simulink model "simulacion_v1"  (R2021b)
settings: Solver=VariableStepAuto  StartTime=0.0  StopTime=100  RelTol=1e-3
undefined symbols (not defined in the file or in its folder): F, h, km, Light, m, MIL, Moderate, s, sigbuilder_block
libraries: slpidlib x19, simulink x18, simulink_extras x15, aerolibconvert2 x4, aerolibwind2 x3, shared6dof x1, sharedtransform x1, sim3dlib x1, uavsim3dlib x1
(part 1 of 3)
settings Model: PacingRate=0.710000  Creator=luisq  LastModifiedBy=luisq
settings SolverCC: AlgebraicLoopSolver=TrustRegion
settings DebuggingCC: SFMachineParentedDataDiag=warning

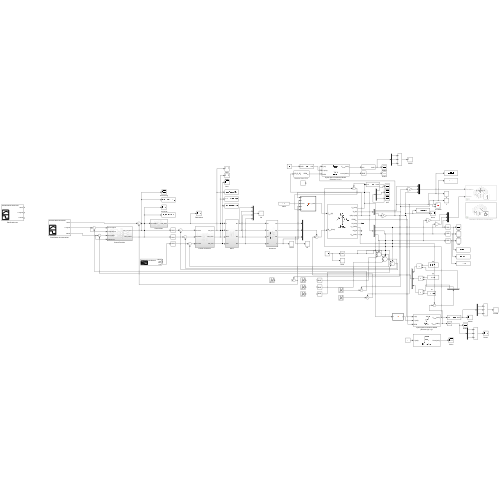
[thumbnail: Simulink's stored preview of the top-level diagram]
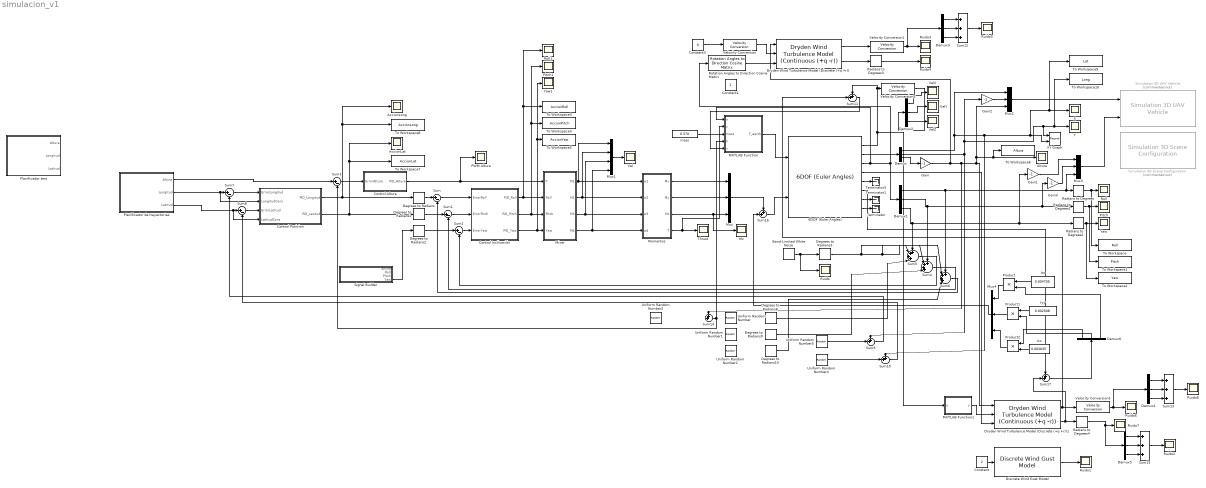
== system simulacion_v1 ==
  6DOF (Euler Angles) : shared6dof/6DOF (Euler Angles)  units=Metric (MKS)  mtype=Fixed  rep=Euler Angles  xme_0=[0 0 0]  Vm_0=[0 0 0]  eul_0=[0 0 0]  pm_0=[0 0 0]  mass_0=0.570  mass_e=0.5  mass_f=2.0  inertia=[0.002635 0 0; 0 0.002508 0; 0 0 0.004705]  inertia_e=eye(3)  inertia_f=2*eye(3)  k_quat=1.0  vre_flag=on  abi_flag=off  aMode=0  xme_statename=''  Vm_statename=''  eul_statename=''  quat_statename=''  pm_statename=''  mass_statename=''
      settings: SourceProductBaseCode=AE,PW,DR,MT,UV,VE
  AccionLat : Scope
  AccionLong : Scope
  Altura : Scope
  Band-Limited White Noise : simulink/Sources/Band-Limited White Noise  Cov=[0.00005]  Ts=0.006  seed=[1165241]
  Constant : Constant  Value=2
  Constant1 : Constant
  Constant3 : Constant  Value=0
  Control Altura : Subsystem
  Control Inclinación : Subsystem
  Control Posicion : Subsystem
  Degrees to Radians{,1..3,8..10} (7 alike) : simulink_extras/Transformations/Degrees to Radians
  Demux{,1..6} (7 alike) : Demux  Outputs=3
  Discrete Wind Gust Model : aerolibwind2/Discrete Wind Gust Model  units=Metric (MKS)  Gx=on  Gy=on  Gz=on  t_0=1  d_m=[100 100 100]  v_m=[2 2 2]
  Dryden Wind Turbulence Model (Discrete (+q +r)) : aerolibwind2/Dryden Wind Turbulence Model  (Continuous (+q -r))  units=Metric (MKS)  spec=MIL-F-8785C  model=Discrete Dryden (+q +r)  W20=15  Wdeg=0  TurbProb=10^-2 - Light  L_high=533.4  Wingspan=10  ts=0.1  Seed=[2753 27856 45178 58756]  T_on=on
  Dryden Wind Turbulence Model (Discrete (+q +r))1 : aerolibwind2/Dryden Wind Turbulence Model  (Continuous (+q -r))  units=Metric (MKS)  spec=MIL-F-8785C  model=Discrete Dryden (+q +r)  W20=1  Wdeg=0  TurbProb=10^-3 - Moderate  L_high=10  Wingspan=20  ts=0.1  Seed=[2753 27856 45178 58756]  T_on=on
  Gain{,1..3} (4 alike) : Gain  Gain=-1
  Ixx : Constant  Value=0.002635
  Iyy : Constant  Value=0.002508
  Izz : Constant  Value=0.004705
  MATLAB Function : MATLAB Function  TreatAsAtomicUnit=on
  MATLAB Function1 : MATLAB Function  TreatAsAtomicUnit=on
  "Mixer " : Subsystem
  Momentos : Subsystem
  Mux{,2..4} (4 alike) : Mux  Inputs=3
  Mux1 : Mux
  Mz : Scope
  PWM Altura : Scope
  Pitch : Scope
  Pitch1 : Scope
  Planificador de trayectorias : Subsystem  Tag=STV Subsys  LoadFcn=sigbuilder_block('load');  StartFcn=sigbuilder_block('start');  StopFcn=sigbuilder_block('stop');  ClipboardFcn=sigbuilder_block('clipboard');  mask(Sigbuilder block){tuvar=[0:10]}
      mask help: Simulink:masks:SigbuilderBlock_MD
      mask init:
      | if ~strcmp(get_param(bdroot(gcbh),'SimulationStatus'),'stopped') tuvar = sigbuilder_block('maskInit'); end
      settings: CopyFcn=sigbuilder_block('copy');  DeleteFcn=sigbuilder_block('delete');  ModelCloseFcn=sigbuilder_block('modelClose');  PreSaveFcn=sigbuilder_block('preSave');  PauseFcn=sigbuilder_block('pause');  ContinueFcn=sigbuilder_block('continue');  NameChangeFcn=sigbuilder_block('namechange');  OpenFcn=sigbuilder_block('open',[438 258 412.5 377.25 ]);  CloseFcn=sigbuilder_block('close');
      mask Display: plot(0, 0, 100, 100,[2, 2, 32, 32, 2], [68, 8, 8, 68, 68],[32, 2], [38, 38], [32, 19, 2],[53, 60, 44], [32, 17, 17, 2],[16, 16, 31, 31]);txt = getActiveGroup(gcbh);text(2, 100, txt,'verticalAlignment', 'top');
  Planificador test : Subsystem  Tag=STV Subsys  LoadFcn=sigbuilder_block('load');  StartFcn=sigbuilder_block('start');  StopFcn=sigbuilder_block('stop');  ClipboardFcn=sigbuilder_block('clipboard');  mask(Sigbuilder block){tuvar=[0:10]}
      mask help: Simulink:masks:SigbuilderBlock_MD
      mask init:
      | if ~strcmp(get_param(bdroot(gcbh),'SimulationStatus'),'stopped') tuvar = sigbuilder_block('maskInit'); end
      settings: CopyFcn=sigbuilder_block('copy');  DeleteFcn=sigbuilder_block('delete');  ModelCloseFcn=sigbuilder_block('modelClose');  PreSaveFcn=sigbuilder_block('preSave');  PauseFcn=sigbuilder_block('pause');  ContinueFcn=sigbuilder_block('continue');  NameChangeFcn=sigbuilder_block('namechange');  OpenFcn=sigbuilder_block('open',[438 258 412.5 377.25 ]);  CloseFcn=sigbuilder_block('close');
      mask Display: plot(0, 0, 100, 100,[2, 2, 32, 32, 2], [68, 8, 8, 68, 68],[32, 2], [38, 38], [32, 19, 2],[53, 60, 44], [32, 17, 17, 2],[16, 16, 31, 31]);txt = getActiveGroup(gcbh);text(2, 100, txt,'verticalAlignment', 'top');
  Product : Product
  Product1 : Product
  Product2 : Product
  Radians to Degrees{,1..4} (5 alike) : simulink_extras/Transformations/Radians to Degrees
  Roll : Scope
  Roll1 : Scope
  Rotation Angles to Direction Cosine Matrix : sharedtransform/Rotation Angles to Direction Cosine Matrix  rotationOrder=ZYX  aMode=aMode
      settings: SourceProductBaseCode=AE,PW,DR,MT,UV,VE
  Ruido{,1..8} (9 alike) : Scope
  Signal Builder : Subsystem  Tag=STV Subsys  LoadFcn=sigbuilder_block('load');  StartFcn=sigbuilder_block('start');  StopFcn=sigbuilder_block('stop');  ClipboardFcn=sigbuilder_block('clipboard');  mask(Sigbuilder block){tuvar=[0:10]}
      mask help: Simulink:masks:SigbuilderBlock_MD
      mask init:
      | if ~strcmp(get_param(bdroot(gcbh),'SimulationStatus'),'stopped') tuvar = sigbuilder_block('maskInit'); end
      settings: CopyFcn=sigbuilder_block('copy');  DeleteFcn=sigbuilder_block('delete');  ModelCloseFcn=sigbuilder_block('modelClose');  PreSaveFcn=sigbuilder_block('preSave');  PauseFcn=sigbuilder_block('pause');  ContinueFcn=sigbuilder_block('continue');  NameChangeFcn=sigbuilder_block('namechange');  OpenFcn=sigbuilder_block('open',[665.25 86.25 550.5 399.75 ]);  CloseFcn=sigbuilder_block('close');
      mask Display: plot(0, 0, 100, 100,[2, 2, 32, 32, 2], [68, 8, 8, 68, 68],[32, 2], [38, 38], [32, 19, 2],[53, 60, 44], [32, 17, 17, 2],[16, 16, 31, 31]);txt = getActiveGroup(gcbh);text(2, 100, txt,'verticalAlignment', 'top');
  Simulation 3D Scene Configuration : sim3dlib/Simulation 3D Scene Configuration  Priority=0  Commented=on  ProjectFormat_internal=Default Scenes  ProjectFormat=Default Scenes  SceneDesc=US city block  ProjectName=G:\MATLAB\R2021b\toolbox\shared\sim3d_projects\automotive_project\UE4\WindowsNoEditor\VehicleSimulation.exe  ScenePath=/Game/Maps/USCityBlock  vehTagList={'Scene Origin';'SimulinkVehicle1'}  vehTag=SimulinkVehicle1  OpVisEn=off  Ts=1/60  EnableWindow=on  EnableWeather=off  SunAltitude=40.0  SunAzimuth=90  clouds=10  wind=1  fog=0  rain=0  sensorTag=MainCamera1  sensorId=1  sensorName=MainCamera1  mountLoc=Origin  offsetFlag=off  tmountOffset=[0, 0, 0]  rmountOffset=[0, 0, 0]  HorizontalResolution=1280  VerticalResolution=720  HorizontalFOV=60  mountPoint=[0 0 0]  mountOrientation=[0 0 0]  aMode=4  ID=1
      settings: SourceProductBaseCode=AE,DR,UV,VE
  Simulation 3D UAV Vehicle : uavsim3dlib/Simulation 3D UAV Vehicle  Priority=-1  Commented=on  Mesh=Quadrotor  MeshPath=/MathWorksUAVContent/UAVs/HexaRotorUAV/HexaRotor.HexaRotor  Color=Black  ActorName=SimulinkVehicle1  InitialTranslation=[0 0 0]  InitialRotation=[0 0 0]  SampleTime=-1  ActorType=SimulinkVehicle  ID=1  aMode=4  ActorTag=SimulinkVehicle1
      settings: SourceProductBaseCode=UV
  Sum{,1..3,7..8} (6 alike) : Sum  Inputs=|+-
  Sum{9..11,14,16..17} (6 alike) : Sum  Inputs=++|
  Sum12 : Sum  Inputs=+++
  Sum13 : Sum  Inputs=+++
  Sum15 : Sum  Inputs=+++
  Sum4 : Sum  Inputs=++++|
  Sum5 : Sum  Inputs=++++|
  Sum6 : Sum  Inputs=++++|
  Terminator : Terminator
  Terminator1 : Terminator
  Terminator3 : Terminator
  Thrust : Scope
  To Workspace : ToWorkspace  VariableName=Roll  SaveFormat=Timeseries  SampleTime=-1
  To Workspace1 : ToWorkspace  VariableName=Pitch  SaveFormat=Timeseries  SampleTime=-1
  To Workspace10 : ToWorkspace  VariableName=Long  SaveFormat=Timeseries  SampleTime=-1
  To Workspace2 : ToWorkspace  VariableName=Yaw  SaveFormat=Timeseries  SampleTime=-1
  To Workspace3 : ToWorkspace  VariableName=AccionRoll  SaveFormat=Timeseries  SampleTime=-1
  To Workspace4 : ToWorkspace  VariableName=AccionPitch  SaveFormat=Timeseries  SampleTime=-1
  To Workspace5 : ToWorkspace  VariableName=AccionYaw  SaveFormat=Timeseries  SampleTime=-1
  To Workspace6 : ToWorkspace  VariableName=Altura  SaveFormat=Timeseries  SampleTime=-1
  To Workspace7 : ToWorkspace  VariableName=AccionLat  SaveFormat=Timeseries  SampleTime=-1
  To Workspace8 : ToWorkspace  VariableName=AccionLong  SaveFormat=Timeseries  SampleTime=-1
  To Workspace9 : ToWorkspace  VariableName=Lat  SaveFormat=Timeseries  SampleTime=-1
  Uniform Random Number : UniformRandomNumber  Minimum=-2.5  Maximum=2.5  Seed=17864  SampleTime=0.006
  Uniform Random Number1 : UniformRandomNumber  Minimum=-2.5  Maximum=2.5  Seed=78834537  SampleTime=0.006
  Uniform Random Number2 : UniformRandomNumber  Minimum=-2.5  Maximum=2.5  Seed=2564558  SampleTime=0.006
  Uniform Random Number3 : UniformRandomNumber  Minimum=-0.6  Maximum=0.6  Seed=418765  SampleTime=0.006
  Uniform Random Number4 : UniformRandomNumber  Minimum=-0.01  Maximum=0.01  Seed=48576  SampleTime=0.006
  Uniform Random Number5 : UniformRandomNumber  Minimum=-0.01  Maximum=0.01  Seed=184832  SampleTime=0.006
  Vel : Scope
  VelX : Scope
  VelY : Scope
  VelZ : Scope
  Velocity Conversion : aerolibconvert2/Velocity Conversion  IU=km/h  OU=m/s
  Velocity Conversion1 : aerolibconvert2/Velocity Conversion  IU=m/s  OU=km/h
  Velocity Conversion3 : aerolibconvert2/Velocity Conversion  IU=m/s  OU=km/h
  Velocity Conversion5 : aerolibconvert2/Velocity Conversion  IU=m/s  OU=km/h
  X : Scope
  XY Graph : Record  FileSettingsInternal="{\"entries\":[{\"content\":{\"excelSettings\":{\"content\":{},\"type\":\"Streamout.ExcelSettings\"}},\"type\":\"Streamout.FileSettingStorage\",\"uuid\":\"2a93f9ce-f61f-4d98-8c9f-4a9fc70b4bb0\"}],\"packageUris\":[\"http://schema.mathworks.com/mf0/streamout_blocks/R2020a\"],\"version\":\"1.0\"}"  Layout=[1 1]  SignalsInternal="{\"entries\":[{\"content\":{\"signals\":[{\"content\":{\"blockPath\":[\"simulacion_v1/XY Graph\"],\"channel\":[],\"dimensions\":[1],\"domain\":\"simulacion_v1/XY Graph\",\"lineColor\":\"#0072bd\",\"plots\":[],\"port\":1,\"sid\":[\"\"],\"signalID\":535,\"signalName\":\"Demux:2\"},\"type\":\"RecordBlkView.Signal\",\"uuid\":\"45a79901-b02e-4be6-b1bb-67b95a6d7ae1\"},{\"content\":{\"blockPath\":[\"simulacion_v1/XY Graph\"],\"channel\":[],\"dimensions\":[1],\"domain\":\"simulacion_v1/XY Graph\",\"lineColor\":\"#d95319\",\"plots\":[],\"port\":2,\"sid\":[\"\"],\"signalID\":539,\"signalName\":\"Demux:1\"},\"type\":\"RecordBlkView.Signal\",\"uuid\":\"d0057eb7-e3a9-49c5-b525-a3b9d954fb19\"}]},\"type\":\"RecordBlkView.InputSignals\",\"uuid\":\"e3ca6051-dc1f-4f56-a0fa-706f4109eb97\"}],\"packageUris\":[\"http://schema.mathworks.com/mf0/streamout_blocks/R2020a\"],\"version\":\"1.0\"}"  CompatibilityTag=XY  st=0.5
  Y : Scope
  Yaw : Scope
  Yaw1 : Scope
  "mass " : Constant  Value=0.570
  wires:
  MATLAB Function/1(F_earth) -> 6DOF (Euler Angles)/1
  Momentos/1(Mx) -> Mux/1
  Momentos/3("Mz ") -> Mz/1, Mux/3
  Momentos/2("My ") -> Mux/2
  "mass "/1 -> MATLAB Function/3(mass)
  6DOF (Euler Angles)/3 -> Demux1/1, Rotation Angles to Direction Cosine Matrix/1, MATLAB Function/1(u)
  6DOF (Euler Angles)/2 -> Demux/1
  Demux/2 -> Sum9/1, XY Graph/1, To Workspace10/1, Y/1, Gain2/1
  Momentos/4(T) -> Thrust/1, MATLAB Function/2(c)
  Demux/3 -> Gain/1
  Demux1/1 -> Sum6/1, Mux3/3, Radians to Degrees/1
  Demux1/3 -> Radians to Degrees2/1, Gain1/1, Sum5/1
  Degrees to Radians/1 -> Sum/1
  Signal Builder/4(Yaw) -> Degrees to Radians2/1
  Degrees to Radians1/1 -> Sum1/1
  Degrees to Radians2/1 -> Sum2/1
  Radians to Degrees/1 -> To Workspace/1, Roll/1
  "Mixer "/1(M1) -> Momentos/1(w1), Mux1/1
  "Mixer "/2("M2 ") -> Momentos/2(w2), Mux1/2
  "Mixer "/3(M3) -> Momentos/3(w3), Mux1/3
  "Mixer "/4(M4) -> Momentos/4(w4), Mux1/4
  Radians to Degrees1/1 -> To Workspace1/1, Pitch/1
  Gain/1 -> Dryden Wind Turbulence Model (Discrete (+q +r))1/1, Mux2/3, To Workspace6/1, Altura/1, Sum14/1, Dryden Wind Turbulence Model (Discrete (+q +r))/1
  Mux1/1 -> Vel/1
  Sum/1 -> Control Inclinación/1(ErrorRoll)
  6DOF (Euler Angles)/1 -> MATLAB Function1/1(u), Velocity Conversion5/1, Sum11/1
  6DOF (Euler Angles)/8 -> Terminator/1
  6DOF (Euler Angles)/7 -> Terminator1/1
  6DOF (Euler Angles)/6 -> Sum17/1
  6DOF (Euler Angles)/5 -> Terminator3/1
  6DOF (Euler Angles)/4 -> Dryden Wind Turbulence Model (Discrete (+q +r))1/3
  Demux2/3 -> VelZ/1
  Radians to Degrees2/1 -> To Workspace2/1, Yaw/1
  Sum1/1 -> Control Inclinación/2(ErrorPitch)
  Sum2/1 -> Control Inclinación/3(ErrorYaw)
  Demux1/2 -> Sum4/1, Gain3/1, Radians to Degrees1/1
  Demux/1 -> Mux2/1, Sum10/1, XY Graph/2, To Workspace9/1, X/1
  Gain2/1 -> Mux2/2
  Band-Limited White Noise/1 -> Ruido/1, Degrees to Radians3/1
  Sum5/1 -> Sum2/2
  Degrees to Radians3/1 -> Sum4/2, Sum5/2, Sum6/2
  Sum4/1 -> Sum1/2
  Sum6/1 -> Sum/2
  Discrete Wind Gust Model/1 -> Ruido1/1
  Constant/1 -> Discrete Wind Gust Model/1
  Demux2/2 -> VelY/1
  Demux2/1 -> VelX/1
  Sum3/1 -> Control Altura/1(ErrorAltura)
  Sum7/1 -> Control Posicion/1(ErrorLongitud)
  Sum8/1 -> Control Posicion/3(ErrorLatitud)
  Sum10/1 -> Sum8/2
  Sum9/1 -> Sum7/2
  Dryden Wind Turbulence Model (Discrete (+q +r))/1 -> Velocity Conversion1/1
  Sum11/1 -> MATLAB Function/5(v)
  Rotation Angles to Direction Cosine Matrix/1 -> Dryden Wind Turbulence Model (Discrete (+q +r))/3
  Dryden Wind Turbulence Model (Discrete (+q +r))/2 -> Radians to Degrees3/1
  Radians to Degrees3/1 -> Ruido4/1
  Constant3/1 -> Velocity Conversion/1
  Velocity Conversion/1 -> Dryden Wind Turbulence Model (Discrete (+q +r))/2
  Velocity Conversion1/1 -> Demux3/1, Ruido3/1
  Demux3/1 -> Sum12/1
  Demux3/2 -> Sum12/2
  Demux3/3 -> Sum12/3
  Sum12/1 -> Ruido5/1
  Velocity Conversion3/1 -> Demux4/1, Ruido6/1
  Demux4/3 -> Sum13/3
  Demux4/1 -> Sum13/1
  MATLAB Function1/1(y) -> Dryden Wind Turbulence Model (Discrete (+q +r))1/2
  Demux4/2 -> Sum13/2
  Sum13/1 -> Ruido8/1
  Dryden Wind Turbulence Model (Discrete (+q +r))1/1 -> Sum11/2, Velocity Conversion3/1
  Velocity Conversion5/1 -> Demux2/1
  Mux2/1 -> Simulation 3D UAV Vehicle/1
  Mux3/1 -> Simulation 3D UAV Vehicle/2
  Gain1/1 -> Mux3/1
  Gain3/1 -> Mux3/2
  Control Altura/1(PID_Altura) -> PWM Altura/1, "Mixer "/1(T)
  Control Inclinación/3(PID_Yaw) -> Yaw1/1, To Workspace5/1, "Mixer "/4(Yaw)
  Control Inclinación/1(PID_Roll) -> Roll1/1, To Workspace3/1, "Mixer "/2(Roll)
  Control Inclinación/2(PID_Pitch) -> Pitch1/1, To Workspace4/1, "Mixer "/3(Pitch)
  Degrees to Radians8/1 -> Sum5/4
  Degrees to Radians9/1 -> Sum4/4
  Degrees to Radians10/1 -> Sum6/4
  Sum14/1 -> MATLAB Function/4(h), Sum3/2
  Control Posicion/1(PID_Longitud) -> Degrees to Radians/1, To Workspace8/1, AccionLong/1
  Control Posicion/2(PID_Latitud) -> Degrees to Radians1/1, AccionLat/1, To Workspace7/1
  Demux5/3 -> Sum15/3
  Demux5/1 -> Sum15/1
  Sum15/1 -> Ruido2/1
  Demux5/2 -> Sum15/2
  Radians to Degrees4/1 -> Ruido7/1, Demux5/1
  Dryden Wind Turbulence Model (Discrete (+q +r))1/2 -> Sum17/2, Radians to Degrees4/1
  Izz/1 -> Product/1
  Ixx/1 -> Product2/2
  Iyy/1 -> Product1/1
  Demux6/1 -> Product2/1
  Demux6/2 -> Product1/2
  Demux6/3 -> Product/2
  Product/1 -> Mux4/1
  Product1/1 -> Mux4/2
  Product2/1 -> Mux4/3
  Mux/1 -> Sum16/1
  Sum16/1 -> 6DOF (Euler Angles)/2
  Mux4/1 -> Sum16/2
  Sum17/1 -> Demux6/1
  Planificador de trayectorias/1(Altura) -> Sum3/1
  Planificador de trayectorias/2(Longitud) -> Control Posicion/2(LongitudCons), Sum7/1
  Planificador de trayectorias/3(Latitud) -> Control Posicion/4(LatitudCons), Sum8/1
  Uniform Random Number5/1 -> Sum9/2
  Uniform Random Number4/1 -> Sum10/2

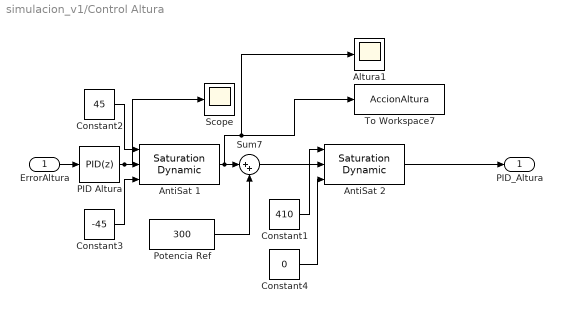
== system simulacion_v1/Control Altura ==
  ErrorAltura : Inport
  Altura1 : Scope
  AntiSat 1 : simulink/Discontinuities/Saturation Dynamic  OutMin=[]  OutMax=[]  OutDataTypeStr=Inherit: Same as second input  OutDataType=fixdt(1, 16)  OutScaling=2^-10  DoSatur=off
  AntiSat 2 : simulink/Discontinuities/Saturation Dynamic  OutMin=[]  OutMax=[]  OutDataTypeStr=Inherit: Same as second input  OutDataType=fixdt(1, 16)  OutScaling=2^-10  DoSatur=off
  Constant1 : Constant  Value=410
  Constant2 : Constant  Value=45
  Constant3 : Constant  Value=-45
  Constant4 : Constant  Value=0
  PID Altura : slpidlib/PID Controller  Controller=PID  Form=Parallel  TimeDomain=Discrete-time  UseExternalTs=off  SampleTime=0.012  IntegratorMethod=Forward Euler  FilterMethod=Forward Euler  ControllerParametersSource=internal  P=9  I=0.8  D=4.5  UseFilter=off  N=100  TunerSelectOption=Transfer Function Based (PID Tuner App)  InitialConditionSource=internal  InitialConditionForIntegrator=0  InitialConditionForFilter=0  DifferentiatorICPrevScaledInput=0  ExternalReset=none  TrackingMode=off  Kt=1  LimitOutput=off  SatLimitsSource=internal  UpperSaturationLimit=inf  LowerSaturationLimit=-inf  LinearizeAsGain=off  AntiWindupMode=none  Kb=1  POutMin=[]  POutMax=[]  IOutMin=[]  IOutMax=[]  DOutMin=[]  DOutMax=[]  NOutMin=[]  NOutMax=[]  SumOutMin=[]  SumOutMax=[]  SaturationOutMin=[]  SaturationOutMax=[]  PParamMin=[]  PParamMax=[]  IParamMin=[]  IParamMax=[]  DParamMin=[]  DParamMax=[]  NParamMin=[]  NParamMax=[]  KbParamMin=[]  KbParamMax=[]  KtParamMin=[]  KtParamMax=[]  KbOutMin=[]  KbOutMax=[]  KtOutMin=[]  KtOutMax=[]  IntegratorOutMin=[]  IntegratorOutMax=[]  FilterOutMin=[]  FilterOutMax=[]  SumI1OutMin=[]  SumI1OutMax=[]  SumI2OutMin=[]  SumI2OutMax=[]  SumI3OutMin=[]  SumI3OutMax=[]  SumI4OutMin=[]  SumI4OutMax=[]  SumDOutMin=[]  SumDOutMax=[]  DifferentiatorOutMin=[]  DifferentiatorOutMax=[]  FilterDiffOutCoefMin=[]  FilterDiffOutCoefMax=[]  ReciprocalOutMin=[]  ReciprocalOutMax=[]  SumDenOutMin=[]  SumDenOutMax=[]  SumNumOutMin=[]  SumNumOutMax=[]  DivideOutMin=[]  DivideOutMax=[]  UdiffTsProdOutMin=[]  UdiffTsProdOutMax=[]  NTsProdOutMin=[]  NTsProdOutMax=[]  UintegralTsProdOutMin=[]  UintegralTsProdOutMax=[]  UngainTsProdOutMin=[]  UngainTsProdOutMax=[]  IntegratorContinuousStateAttributes=''  IntegratorStateMustResolveToSignalObject=off  IntegratorRTWStateStorageClass=Auto  FilterContinuousStateAttributes=''  FilterStateMustResolveToSignalObject=off  FilterRTWStateStorageClass=Auto  ParallelPVariant=InternalParameters  IdealPVariant=Disabled  IVariant=InternalParameters  DVariant=InternalParameters  IntegratorVariant=Discrete  SatVariant=Disabled  AWVariant=Passthrough  PCopyVariant=Disabled  TRVariant=Disabled  FdbkBlocksVariant=Forward  IdealPFdbkVariant=Disabled  SatFdbkVariant=Disabled  DerivativeFilterVariant=Differentiator  NVariant=Passthrough  NCopyVariant=Disabled_SignalSpec  FilterICVariant=InternalICsDifferentiator  IntegratorICVariant=InternalICs  ExternalResetVariant=Disabled  TRSumVariant=Passthrough  SumFdbkVariant=Disabled  SumVariant=Sum_PID  TsampFilterVariant=InternalTs  TsampNgainVariant=Passthrough  TsampIntegralVariant=Passthrough  ExternalSaturationOutDataTypeStr=Inherit: Same as second input
  Potencia Ref : Constant  Value=300
  Scope : Scope
  Sum7 : Sum  Inputs=|++
  To Workspace7 : ToWorkspace  VariableName=AccionAltura  SaveFormat=Timeseries  SampleTime=-1
  PID_Altura : Outport
  wires:
  Potencia Ref/1 -> Sum7/2
  Constant3/1 -> AntiSat 1/3
  AntiSat 1/1 -> Altura1/1, To Workspace7/1, Sum7/1
  PID Altura/1 -> Scope/1, AntiSat 1/2
  Constant2/1 -> AntiSat 1/1
  ErrorAltura/1 -> PID Altura/1
  Sum7/1 -> AntiSat 2/2
  AntiSat 2/1 -> PID_Altura/1
  Constant1/1 -> AntiSat 2/1
  Constant4/1 -> AntiSat 2/3
